simulink model "normal_forces_edite"  (R2015a)
settings: Solver=ode45  StartTime=0.0  StopTime=10.0  RelTol=1e-3
undefined symbols (not defined in the file or in its folder): magnitude
settings Model: Creator=BML  LastModifiedBy=BML

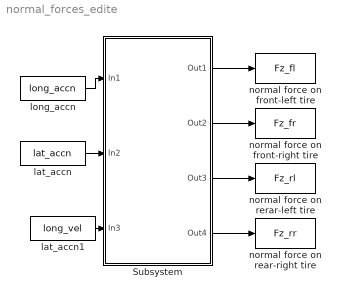
== system normal_forces_edite ==
  Subsystem : Subsystem
  lat_accn : FromWorkspace  VariableName=lat_accn  SampleTime=0
  lat_accn1 : FromWorkspace  VariableName=long_vel  SampleTime=0
  long_accn : FromWorkspace  VariableName=long_accn  SampleTime=0
  normal force on front-left tire : ToWorkspace  VariableName=Fz_fl  SaveFormat=Timeseries  SampleTime=-1
  normal force on front-right tire : ToWorkspace  VariableName=Fz_fr  SaveFormat=Timeseries  SampleTime=-1
  normal force on rear-right tire : ToWorkspace  VariableName=Fz_rr  SaveFormat=Timeseries  SampleTime=-1
  normal force on rerar-left tire : ToWorkspace  VariableName=Fz_rl  SaveFormat=Timeseries  SampleTime=-1
  wires:
  long_accn/1 -> Subsystem/1(In1)
  lat_accn/1 -> Subsystem/2(In2)
  Subsystem/1(Out1) -> normal force on front-left tire/1
  Subsystem/2(Out2) -> normal force on front-right tire/1
  Subsystem/3(Out3) -> normal force on rerar-left tire/1
  Subsystem/4(Out4) -> normal force on rear-right tire/1
  lat_accn1/1 -> Subsystem/3(In3)

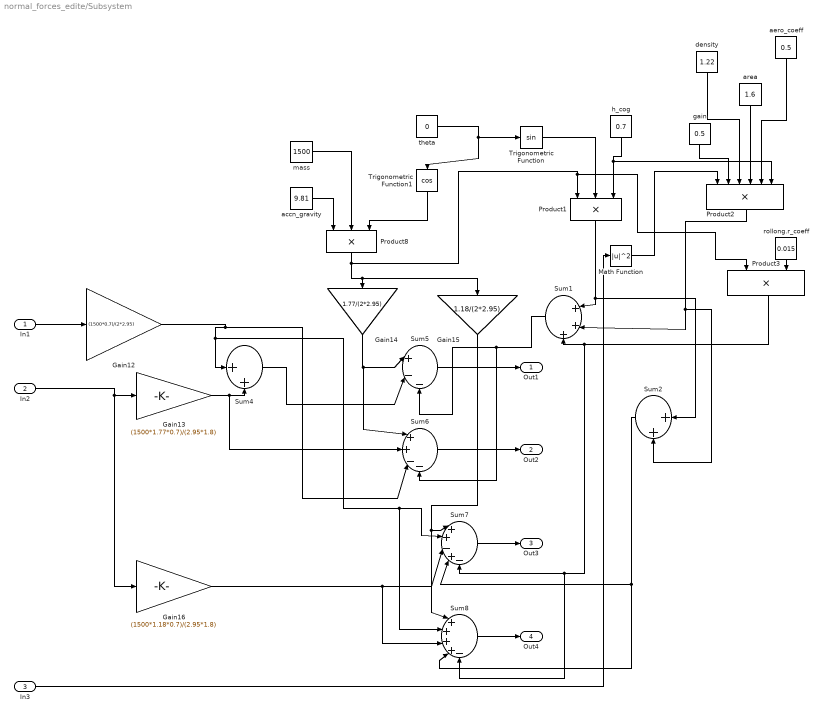
== system normal_forces_edite/Subsystem ==
  In1 : Inport
  In2 : Inport  Port=2
  In3 : Inport  Port=3
  Gain12 : Gain  Gain=(1500*0.7)/(2*2.95)
  Gain13 : Gain  Gain=(1500*1.77*0.7)/(2.95*1.8)
  Gain14 : Gain  Gain=1.77/(2*2.95)
  Gain15 : Gain  Gain=1.18/(2*2.95)
  Gain16 : Gain  Gain=(1500*1.18*0.7)/(2.95*1.8)
  Math Function : Math  Operator=magnitude^2  SaturateOnIntegerOverflow=on
  Product1 : Product  Inputs=3
  Product2 : Product  Inputs=6
  Product3 : Product
  Product8 : Product  Inputs=3
  Sum1 : Sum  Inputs=|+++
  Sum2 : Sum  Inputs=|++
  Sum4 : Sum  Inputs=|++
  Sum5 : Sum  Inputs=|+--
  Sum6 : Sum  Inputs=|++--
  Sum7 : Sum  Inputs=|++-+-
  Sum8 : Sum  Inputs=|++++-
  Trigonometric Function : Trigonometry
  Trigonometric Function1 : Trigonometry  Operator=cos
  "accn_gravity " : Constant  Value=9.81
  "aero_coeff " : Constant  Value=0.5
  "area " : Constant  Value=1.6
  "density " : Constant  Value=1.22
  gain : Constant  Value=0.5
  "h_cog " : Constant  Value=0.7
  mass : Constant  Value=1500
  "rollong.r_coeff " : Constant  Value=0.015
  theta : Constant  Value=0
  Out1 : Outport
  Out2 : Outport  Port=2
  Out3 : Outport  Port=3
  Out4 : Outport  Port=4
  wires:
  Gain12/1 -> Sum4/1, Sum8/2, Sum7/2, Sum6/3
  Gain15/1 -> Sum8/1, Sum7/1
  Gain16/1 -> Sum8/3, Sum7/3
  Sum7/1 -> Out3/1
  In2/1 -> Gain16/1, Gain13/1
  Gain13/1 -> Sum6/2, Sum4/2
  Sum5/1 -> Out1/1
  Sum6/1 -> Out2/1
  Sum4/1 -> Sum5/2
  In1/1 -> Gain12/1
  mass/1 -> Product8/2
  Gain14/1 -> Sum5/1, Sum6/1
  Sum8/1 -> Out4/1
  Product8/1 -> Product3/1, Product1/1, Gain15/1, Gain14/1
  "accn_gravity "/1 -> Product8/1
  theta/1 -> Trigonometric Function1/1, Trigonometric Function/1
  "h_cog "/1 -> Product2/6, Product1/3
  Trigonometric Function/1 -> Product1/2
  In3/1 -> Math Function/1
  Math Function/1 -> Product2/1
  gain/1 -> Product2/2
  "density "/1 -> Product2/3
  "area "/1 -> Product2/4
  "aero_coeff "/1 -> Product2/5
  Trigonometric Function1/1 -> Product8/3
  "rollong.r_coeff "/1 -> Product3/2
  Product1/1 -> Sum2/1, Sum1/1
  Product2/1 -> Sum2/2, Sum1/2
  Product3/1 -> Sum8/5, Sum7/5, Sum1/3
  Sum1/1 -> Sum6/4, Sum5/3
  Sum2/1 -> Sum8/4, Sum7/4
